simulink model "sim_car_gps_x"  (R2022b)
settings: Solver=VariableStepAuto  StartTime=0.0  StopTime=200  RelTol=1e-3
values from neighbouring files (symbols this model uses):
  A = rand(4,4)    [car_gps_x.m]    (also in car_gps_xv.m = [1, Ts, 0.5*Ts^2, 0, 0,  0)
  C = rand(2,4)    [car_gps_x.m]    (also in car_gps_xv.m = [1, 0, 0, 0, 0, 0)
  fgps = 10    [car_gps_x.m]    (also in car_gps_xv.m)
  Kf = Kf_t'    [car_gps_x.m]    (also in car_gps_xv.m)
  Ts = 1/fgps    (= 0.1)    [car_gps_x.m]    (also in car_gps_xv.m)
  xo_hat = [2 0 2 0]'    [car_gps_x.m]    (also in car_gps_xv.m = [2 0 0 2 0 0]')
libraries: simulink x4
settings Model: Creator=ricardoaguilera  LastModifiedBy=lucie
settings SolverCC: AlgebraicLoopSolver=TrustRegion
settings DataIOCC: ReturnWorkspaceOutputs=off
settings DebuggingCC: UnconnectedInputMsg=warning  UnconnectedOutputMsg=warning  UnconnectedLineMsg=warning  SFMachineParentedDataDiag=warning  ArithmeticOperatorsInVariantConditions=warning
settings ModelReferenceCC: EnableRefExpFcnMdlSchedulingChecks=on
settings SFSimCC: CustomCodeUndefinedFunction=UseInterfaceOnly
settings RTWCC: DLArmComputeVersion=19.05

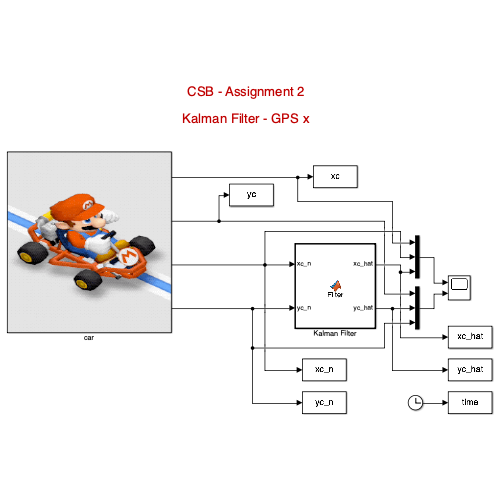
[thumbnail: Simulink's stored preview of the top-level diagram]
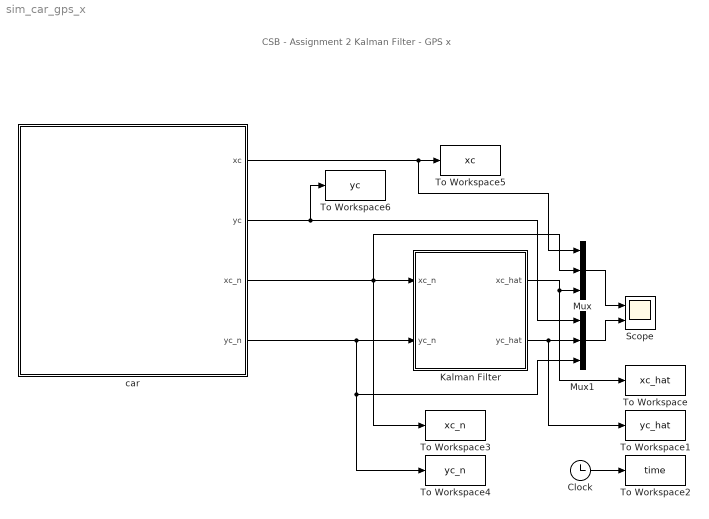
== system sim_car_gps_x ==
  note: CSB - Assignment 2
      |
      | Kalman Filter - GPS x
  Clock : Clock
  Kalman Filter : MATLAB Function  TreatAsAtomicUnit=on  SystemSampleTime=Ts
  Mux : Mux  Inputs=3
  Mux1 : Mux  Inputs=3
  Scope : Scope  NumInputPorts=2
  To Workspace : ToWorkspace  VariableName=xc_hat  SampleTime=Ts
  To Workspace1 : ToWorkspace  VariableName=yc_hat  SampleTime=Ts
  To Workspace2 : ToWorkspace  VariableName=time  SampleTime=Ts
  To Workspace3 : ToWorkspace  VariableName=xc_n  SampleTime=Ts
  To Workspace4 : ToWorkspace  VariableName=yc_n  SampleTime=Ts
  To Workspace5 : ToWorkspace  VariableName=xc  SampleTime=Ts
  To Workspace6 : ToWorkspace  VariableName=yc  SampleTime=Ts
  car : Subsystem
      mask Display: image('$imagefile'); % Use "Edit Image" on toolstrip to change.
  wires:
  Kalman Filter/1(xc_hat) -> To Workspace/1, Mux/3
  Kalman Filter/2(yc_hat) -> To Workspace1/1, Mux1/2
  car/2(yc) -> To Workspace6/1, Mux1/1
  Mux1/1 -> Scope/2
  car/1(xc) -> To Workspace5/1, Mux/1
  Clock/1 -> To Workspace2/1
  car/4(yc_n) -> To Workspace4/1, Mux1/3, Kalman Filter/2(yc_n)
  car/3(xc_n) -> Mux/2, To Workspace3/1, Kalman Filter/1(xc_n)
  Mux/1 -> Scope/1

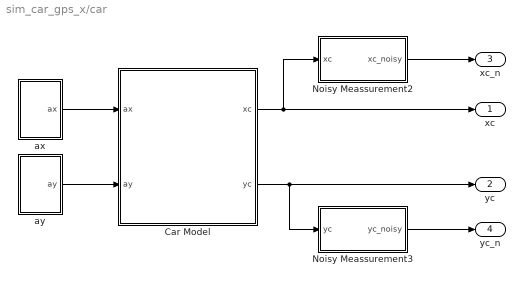
== system sim_car_gps_x/car ==
  Car Model : MATLAB Function  TreatAsAtomicUnit=on  SystemSampleTime=0.1
  Noisy Meassurement2 : Subsystem
  Noisy Meassurement3 : Subsystem
  "ax " : Subsystem
  "ay " : Subsystem
  xc : Outport  VectorParamsAs1DForOutWhenUnconnected=off
  yc : Outport  Port=2  VectorParamsAs1DForOutWhenUnconnected=off
  xc_n : Outport  Port=3  VectorParamsAs1DForOutWhenUnconnected=off
  yc_n : Outport  Port=4  VectorParamsAs1DForOutWhenUnconnected=off
  wires:
  "ax "/1(ax) -> Car Model/1(ax)
  Noisy Meassurement3/1(yc_noisy) -> yc_n/1
  Noisy Meassurement2/1(xc_noisy) -> xc_n/1
  "ay "/1(ay) -> Car Model/2(ay)
  Car Model/1(xc) -> Noisy Meassurement2/1(xc), xc/1
  Car Model/2(yc) -> Noisy Meassurement3/1(yc), yc/1

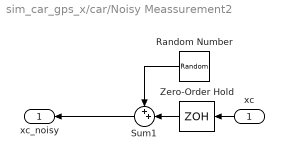
== system sim_car_gps_x/car/Noisy Meassurement2 ==
  xc : Inport
  Random Number : RandomNumber  Variance=7  Seed=1  SampleTime=Ts
  Sum1 : Sum  Inputs=++|
  Zero-Order Hold : ZeroOrderHold  SampleTime=1/fgps
  xc_noisy : Outport  VectorParamsAs1DForOutWhenUnconnected=off
  wires:
  xc/1 -> Zero-Order Hold/1
  Zero-Order Hold/1 -> Sum1/2
  Random Number/1 -> Sum1/1
  Sum1/1 -> xc_noisy/1

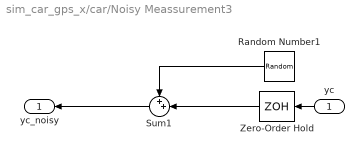
== system sim_car_gps_x/car/Noisy Meassurement3 ==
  yc : Inport
  Random Number1 : RandomNumber  Variance=11  Seed=-1  SampleTime=Ts
  Sum1 : Sum  Inputs=++|
  Zero-Order Hold : ZeroOrderHold  SampleTime=1/fgps
  yc_noisy : Outport  VectorParamsAs1DForOutWhenUnconnected=off
  wires:
  yc/1 -> Zero-Order Hold/1
  Sum1/1 -> yc_noisy/1
  Random Number1/1 -> Sum1/1
  Zero-Order Hold/1 -> Sum1/2

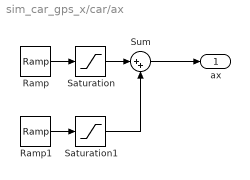
== system sim_car_gps_x/car/ax  ==
  Ramp : simulink/Sources/Ramp  slope=30  start=10  InitialOutput=0
  Ramp1 : simulink/Sources/Ramp  slope=-100  start=20  InitialOutput=0
  Saturation : Saturate  UpperLimit=100  LowerLimit=0
  Saturation1 : Saturate  UpperLimit=1  LowerLimit=-90
  Sum : Sum  Inputs=|++
  ax : Outport  VectorParamsAs1DForOutWhenUnconnected=off
  wires:
  Ramp/1 -> Saturation/1
  Sum/1 -> ax/1
  Ramp1/1 -> Saturation1/1
  Saturation1/1 -> Sum/2
  Saturation/1 -> Sum/1

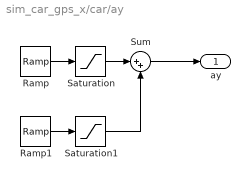
== system sim_car_gps_x/car/ay  ==
  Ramp : simulink/Sources/Ramp  slope=500  start=35  InitialOutput=0
  Ramp1 : simulink/Sources/Ramp  slope=-50  start=40  InitialOutput=0
  Saturation : Saturate  UpperLimit=400  LowerLimit=0
  Saturation1 : Saturate  UpperLimit=0  LowerLimit=-400
  Sum : Sum  Inputs=|++
  ay : Outport  VectorParamsAs1DForOutWhenUnconnected=off
  wires:
  Ramp/1 -> Saturation/1
  Sum/1 -> ay/1
  Ramp1/1 -> Saturation1/1
  Saturation/1 -> Sum/1
  Saturation1/1 -> Sum/2

== matlab function sim_car_gps_x/car/Car Model ==
  data: ax input; xc output; ay input; yc output
function [xc, yc] = fnc(ax, ay)
    [xc,yc] = car_xy_model(ax,ay);
end

== matlab function sim_car_gps_x/Kalman Filter ==
  data: xc_n input; yc_n input; A parameter; C parameter; xc_hat output; Kf parameter; yc_hat output; xo_hat parameter
function [xc_hat,yc_hat] = Filter(xc_n, yc_n, A, C, Kf,xo_hat)

%% Use persistent for variables that require memory
persistent x_hat_k      % Present state estimate 
    if isempty(x_hat_k) 
        x_hat_k = xo_hat;  % State estimate initialization
    end

persistent x_hat_k1         % Next-step state estimate
    if isempty(x_hat_k1)
        x_hat_k1 = xo_hat; % State estimate initialization
    end

%% Filter update 
x_hat_k=x_hat_k1;
%% Measurements

y_k=zeros(2,1);     % To create the output vector (required by Matlab)
y_k=[xc_n yc_n]';

%%  Steady-State Kalman Filter
% Implement here your kalman filter

y_hat_k=C*x_hat_k;

x_hat_k = A * x_hat_k + Kf*(y_k - y_hat_k);


xc_hat = x_hat_k;
yc_hat = C*x_hat_k;
